simulink model "assignment_2_simulink"  (R2023a)
settings: Solver=VariableStepAuto  StartTime=0.0  StopTime=10.0  RelTol=1e-3
settings Model: Creator=chowd  LastModifiedBy=chowd

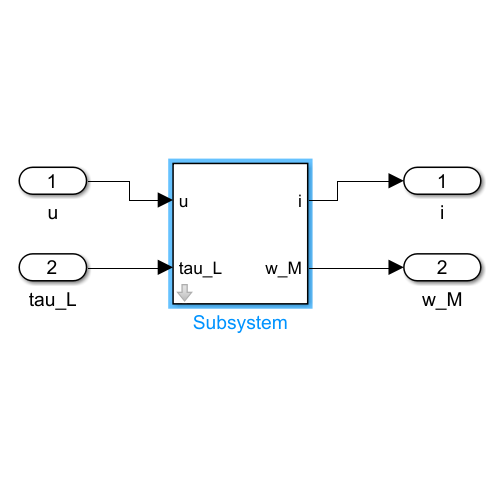
[thumbnail: Simulink's stored preview of the top-level diagram]
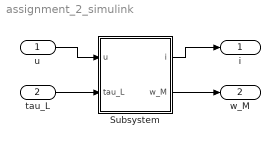
== system assignment_2_simulink ==
  u : Inport
  tau_L : Inport  Port=2
  Subsystem : Subsystem  mask{R=0, L=0, k=0, J=0}
      mask prompts: R "R (ohm)"; L "L (H)"; k "k (Vs)"; J "J (kgm^2)"
  i : Outport
  w_M : Outport  Port=2
  wires:
  u/1 -> Subsystem/1(u)
  tau_L/1 -> Subsystem/2(tau_L)
  Subsystem/1(i) -> i/1
  Subsystem/2(w_M) -> w_M/1

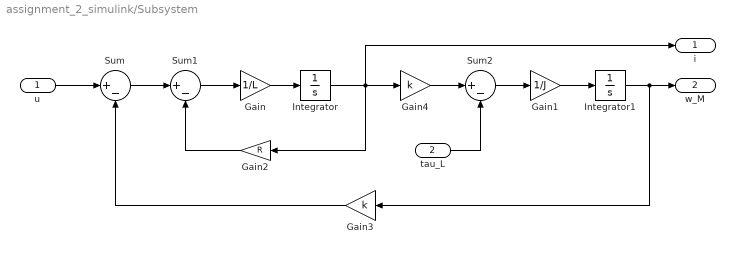
== system assignment_2_simulink/Subsystem ==
  u : Inport
  tau_L : Inport  Port=2
  Gain : Gain  Gain=1/L
  Gain1 : Gain  Gain=1/J
  Gain2 : Gain  Gain=R
  Gain3 : Gain  Gain=k
  Gain4 : Gain  Gain=k
  Integrator : Integrator
  Integrator1 : Integrator
  Sum : Sum  Inputs=|+-
  Sum1 : Sum  Inputs=|+-
  Sum2 : Sum  Inputs=|+-
  i : Outport
  w_M : Outport  Port=2
  wires:
  Gain/1 -> Integrator/1
  Sum2/1 -> Gain1/1
  Sum/1 -> Sum1/1
  u/1 -> Sum/1
  Integrator/1 -> i/1, Gain4/1, Gain2/1
  Sum1/1 -> Gain/1
  Gain2/1 -> Sum1/2
  Gain3/1 -> Sum/2
  tau_L/1 -> Sum2/2
  Integrator1/1 -> w_M/1, Gain3/1
  Gain4/1 -> Sum2/1
  Gain1/1 -> Integrator1/1
